simulink subsystem "arm_format"  (R2024a)
settings: Solver=VariableStepAuto  StartTime=0.0  StopTime=10.0  RelTol=1e-3
settings Model: Creator=gurt1  LastModifiedBy=gurt1

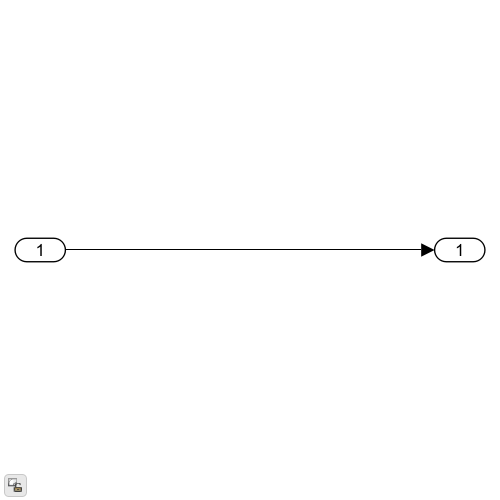
[thumbnail: Simulink's stored preview of the top-level diagram]
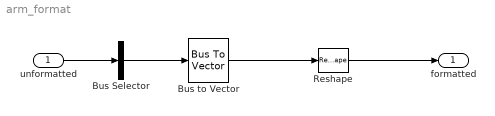
== system arm_format ==
  unformatted : Inport
  Bus Selector : BusSelector  OutputSignals=arm,dt_arm  OutputAsBus=on
  Bus to Vector : BusToVector
  Reshape : Reshape
  formatted : Outport
  wires:
  unformatted/1 -> Bus Selector/1
  Bus Selector/1 -> Bus to Vector/1
  Bus to Vector/1 -> Reshape/1
  Reshape/1 -> formatted/1
